simulink model "controle_malha_fechada_arduino"  (R2024b)
settings: Solver=ode4  StartTime=0.0  StopTime=inf  FixedStep=1e-3  RelTol=1e-3
libraries: arduinolib x6, simulink x1
settings Model: Creator=caioc  LastModifiedBy=helenabrener
settings DebuggingCC: UnconnectedInputMsg=warning  UnconnectedOutputMsg=warning  UnconnectedLineMsg=warning
settings ModelReferenceCC: EnableRefExpFcnMdlSchedulingChecks=on
settings RTWCC: GPUComputeCapability=3.5  DLArmComputeVersion=19.05

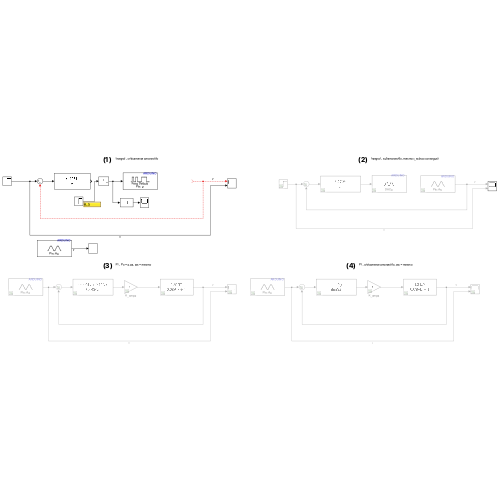
[thumbnail: Simulink's stored preview of the top-level diagram]
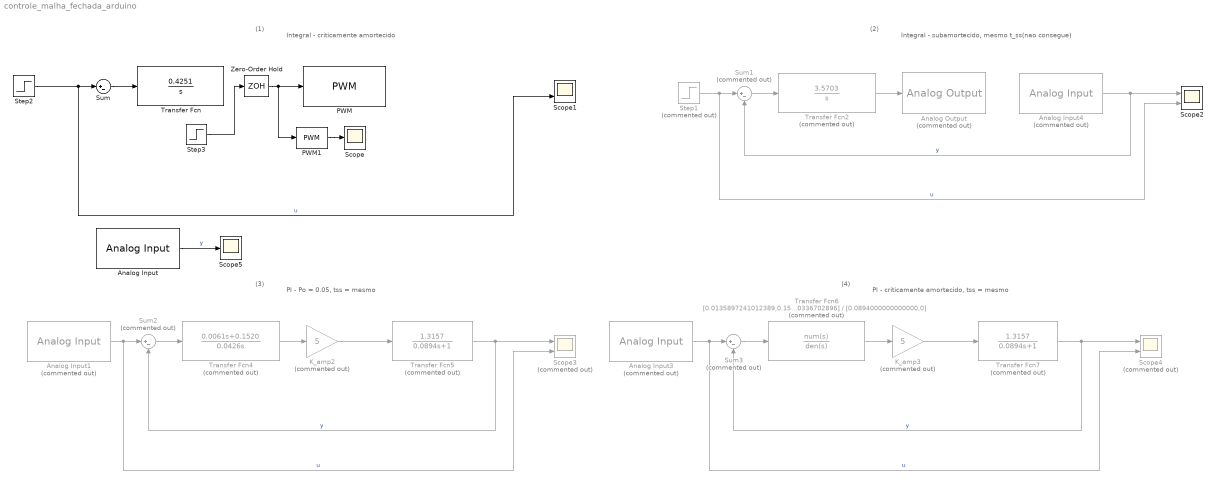
== system controle_malha_fechada_arduino ==
  note: Integral - criticamente amortecido
  note: (1)
  note: (2)
  note: Integral - subamortecido, mesmo t_ss(nao consegue)
  note: (3)
  note: PI - Po = 0.05, tss = mesmo
  note: (4)
  note: PI - criticamente amortecido, tss = mesmo
  Analog Input : arduinolib/Analog Input  pinNumber=4  ReadResultsOnly=off  ConversionTriggerSource=Software  ExternalTriggerType=uint32( 0 )  OutputDataType=uint16  EnableConversionCompleteNotify=off  EnableOuputStatus=off  SampleTime=-1  blockPlatform=arduino
  Analog Input1 : arduinolib/Analog Input  Commented=on  pinNumber=4  ReadResultsOnly=off  ConversionTriggerSource=Software  ExternalTriggerType=uint32( 0 )  OutputDataType=uint16  EnableConversionCompleteNotify=off  EnableOuputStatus=off  SampleTime=-1  blockPlatform=arduino
  Analog Input3 : arduinolib/Analog Input  Commented=on  pinNumber=4  ReadResultsOnly=off  ConversionTriggerSource=Software  ExternalTriggerType=uint32( 0 )  OutputDataType=uint16  EnableConversionCompleteNotify=off  EnableOuputStatus=off  SampleTime=-1  blockPlatform=arduino
  Analog Input4 : arduinolib/Analog Input  Commented=on  pinNumber=5  ReadResultsOnly=off  ConversionTriggerSource=Software  ExternalTriggerType=uint32( 0 )  OutputDataType=uint16  EnableConversionCompleteNotify=off  EnableOuputStatus=off  SampleTime=-1  blockPlatform=arduino
  Analog Output : arduinolib/Analog Output  Commented=on  blockPlatform=ARDUINO  DACpin=DAC0
  K_amp2 : Gain  Commented=on  Gain=5
  K_amp3 : Gain  Commented=on  Gain=5
  PWM : arduinolib/PWM  pinNumber=2  frequencyType=Default  desiredFrequency=490.2  achievableFrequency=490.2
  PWM1 : simulink/Discontinuities/PWM  DisableCoverage=on  Period=1  InitialDelay=0  DisallowZeroDutyCycle=off  RunAtFixedTimeIntervals=on  SampleTime=0.1
  Scope : Scope
  Scope1 : Scope  NumInputPorts=2
  Scope2 : Scope  NumInputPorts=2
  Scope3 : Scope  Commented=on  NumInputPorts=2
  Scope4 : Scope  Commented=on  NumInputPorts=2
  Scope5 : Scope
  Step1 : Step  Commented=on  Time=0  After=10  SampleTime=0
  Step2 : Step  Time=0  After=10  SampleTime=0
  Step3 : Step  Time=0  After=0.5  SampleTime=0
  Sum : Sum  Inputs=|+-
  Sum1 : Sum  Commented=on  Inputs=|+-
  Sum2 : Sum  Commented=on  Inputs=|+-
  Sum3 : Sum  Commented=on  Inputs=|+-
  Transfer Fcn : TransferFcn  Numerator=0.4251  Denominator=[1 0]
  Transfer Fcn2 : TransferFcn  Commented=on  Numerator=3.5703  Denominator=[1 0]
  Transfer Fcn4 : TransferFcn  Commented=on  Numerator=[0.0061 0.1520]  Denominator=[0.0426 0]
  Transfer Fcn5 : TransferFcn  Commented=on  Numerator=[1.3157]  Denominator=[0.0894 1]
  Transfer Fcn6 : TransferFcn  Commented=on  Numerator=[0.0135897241012389,0.152010336702896]  Denominator=[0.0894000000000000,0]
  Transfer Fcn7 : TransferFcn  Commented=on  Numerator=[1.3157]  Denominator=[0.0894 1]
  Zero-Order Hold : ZeroOrderHold  SampleTime=-1
  wires:
  ? -> Sum/2, Scope1/1  "y"
  Step2/1 -> Scope1/2, Sum/1  "u"
  Sum/1 -> Transfer Fcn/1
  Step3/1 -> Zero-Order Hold/1
  Sum1/1 -> Transfer Fcn2/1
  Analog Input4/1 -> Sum1/2, Scope2/1  "y"
  Transfer Fcn2/1 -> Analog Output/1
  Step1/1 -> Sum1/1, Scope2/2  "u"
  Sum2/1 -> Transfer Fcn4/1
  K_amp2/1 -> Transfer Fcn5/1
  Transfer Fcn5/1 -> Sum2/2, Scope3/1  "y"
  Transfer Fcn4/1 -> K_amp2/1
  Analog Input1/1 -> Sum2/1, Scope3/2  "u"
  Analog Input3/1 -> Sum3/1, Scope4/2  "u"
  K_amp3/1 -> Transfer Fcn7/1
  Sum3/1 -> Transfer Fcn6/1
  Transfer Fcn7/1 -> Sum3/2, Scope4/1  "y"
  Transfer Fcn6/1 -> K_amp3/1
  Zero-Order Hold/1 -> PWM1/1, PWM/1
  PWM1/1 -> Scope/1
  Analog Input/1 -> Scope5/1  "y"
